simulink model "ActuatorModel"  (R2020a)
settings: Solver=VariableStepAuto  StartTime=0.0  StopTime=10.0  RelTol=1e-3
values from neighbouring files (symbols this model uses):
  SA_Gain = A_Max/X_Max    (= 16)    [ActuatorModelParams.m]
libraries: fl_lib x34, nesl_utility x4, sdl_lib x1, SignalEditorBlockLib x1
(part 2 of 2)

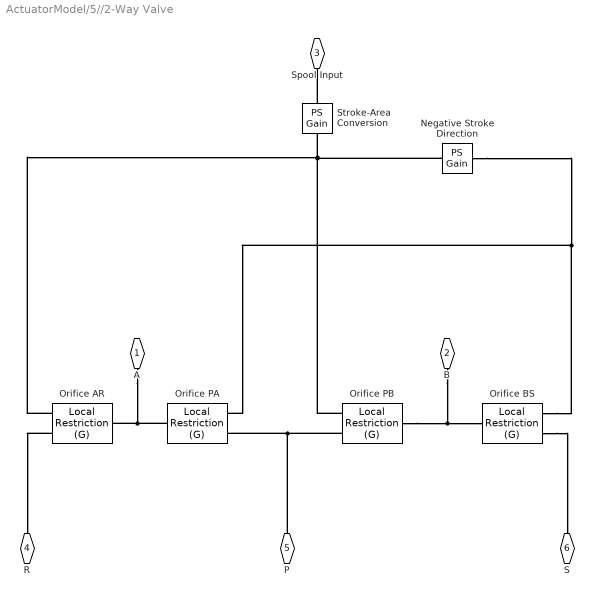
== system ActuatorModel/5//2-Way Valve ==
  Negative Stroke Direction : fl_lib/Physical Signals/Functions/PS Gain  gain=-1
  Orifice AR : fl_lib/Gas/Elements/Local Restriction (G)  restriction_type=foundation.enum.restriction_type.variable  restriction_area=1e-3 m^2  min_area=AR_MinArea in^2  max_area=AR_MaxArea mm^2  area=AR_OriArea in^2  Cd=AR_Cd  B_lam=0.999
      settings: SourceProductBaseCode=SS  InternalSimscapePortConfiguration="{\"Bottom\":[],\"Left\":[{\"id\":\"A\",\"label\":\"A\",\"type\":\"foundation.gas.gas\"},{\"id\":\"area_in\",\"label\":\"AR\",\"type\":\"input\"}],\"Right\":[{\"id\":\"B\",\"label\":\"B\",\"type\":\"foundation.gas.gas\"}],\"Top\":[]}"
  Orifice BS : fl_lib/Gas/Elements/Local Restriction (G)  restriction_type=foundation.enum.restriction_type.variable  restriction_area=1e-3 m^2  min_area=BS_MinArea in^2  max_area=BS_MaxArea mm^2  area=BS_OriArea in^2  Cd=BS_Cd  B_lam=0.999
      settings: SourceProductBaseCode=SS  InternalSimscapePortConfiguration="{\"Bottom\":[],\"Left\":[{\"id\":\"A\",\"label\":\"A\",\"type\":\"foundation.gas.gas\"},{\"id\":\"area_in\",\"label\":\"AR\",\"type\":\"input\"}],\"Right\":[{\"id\":\"B\",\"label\":\"B\",\"type\":\"foundation.gas.gas\"}],\"Top\":[]}"
  Orifice PA : fl_lib/Gas/Elements/Local Restriction (G)  restriction_type=foundation.enum.restriction_type.variable  restriction_area=1e-3 m^2  min_area=PA_MinArea in^2  max_area=PA_MaxArea mm^2  area=PA_OriArea in^2  Cd=PA_Cd  B_lam=0.999
      settings: SourceProductBaseCode=SS  InternalSimscapePortConfiguration="{\"Bottom\":[],\"Left\":[{\"id\":\"A\",\"label\":\"A\",\"type\":\"foundation.gas.gas\"},{\"id\":\"area_in\",\"label\":\"AR\",\"type\":\"input\"}],\"Right\":[{\"id\":\"B\",\"label\":\"B\",\"type\":\"foundation.gas.gas\"}],\"Top\":[]}"
  Orifice PB : fl_lib/Gas/Elements/Local Restriction (G)  restriction_type=foundation.enum.restriction_type.variable  restriction_area=1e-3 m^2  min_area=PB_MinArea in^2  max_area=PB_MaxArea mm^2  area=PB_OriArea in^2  Cd=PB_Cd  B_lam=0.999
      settings: SourceProductBaseCode=SS  InternalSimscapePortConfiguration="{\"Bottom\":[],\"Left\":[{\"id\":\"A\",\"label\":\"A\",\"type\":\"foundation.gas.gas\"},{\"id\":\"area_in\",\"label\":\"AR\",\"type\":\"input\"}],\"Right\":[{\"id\":\"B\",\"label\":\"B\",\"type\":\"foundation.gas.gas\"}],\"Top\":[]}"
  Stroke-Area Conversion : fl_lib/Physical Signals/Functions/PS Gain  gain=SA_Gain
  A : PMIOPort  Side=Left
  B : PMIOPort  Port=2  Side=Left
  Spool Input : PMIOPort  Port=3  Side=Left
  R : PMIOPort  Port=4  Side=Right
  P : PMIOPort  Port=5  Side=Right
  S : PMIOPort  Port=6  Side=Right
  connections:
  Orifice PA/RConn1 -- A/RConn1 -- Orifice AR/RConn1
  Negative Stroke Direction/RConn1 -- Orifice PA/LConn2 -- Orifice BS/LConn2
  Orifice BS/LConn1 -- S/RConn1
  Negative Stroke Direction/LConn1 -- Orifice PB/LConn2 -- Orifice AR/LConn2 -- Stroke-Area Conversion/RConn1
  Orifice PB/LConn1 -- Orifice PA/LConn1 -- P/RConn1
  Orifice PB/RConn1 -- B/RConn1 -- Orifice BS/RConn1
  Stroke-Area Conversion/LConn1 -- Spool Input/RConn1
  Orifice AR/LConn1 -- R/RConn1

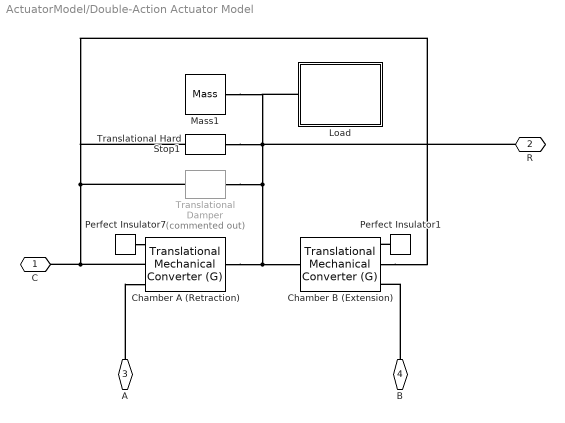
== system ActuatorModel/Double-Action Actuator Model ==
  Chamber A (Retraction) : fl_lib/Gas/Elements/Translational Mechanical Converter (G)  mech_orientation=simscape.enum.posneg.negative  interface_area=ChA_InterfaceArea in^2  length_init=ChA_InitialDisplacement in  dead_volume=ChA_DeadVol in^3  area_A=ChA_PortArea in^2  environment_spec=foundation.enum.pressure_spec.atmospheric  environment_pressure=0.101325 MPa  p_I_specify=off  p_I_priority=High  p_I=0.101325 MPa  p_I_nominal_specify=off  p_I_nominal_unit=MPa  p_I_nominal_value=1  T_I_specify=off  T_I_priority=High  T_I=293.15 K  T_I_nominal_specify=off  T_I_nominal_unit=K  T_I_nominal_value=1  rho_converter_specify=off  rho_converter_priority=None  rho_converter=1.2 kg/m^3  rho_converter_nominal_specify=off  rho_converter_nominal_unit=kg/m^3  rho_converter_nominal_value=1
      settings: SourceProductBaseCode=SS  InternalSimscapePortConfiguration="{\"Bottom\":[],\"Left\":[{\"id\":\"A\",\"label\":\"A\",\"type\":\"foundation.gas.gas\"},{\"id\":\"C\",\"label\":\"C\",\"type\":\"foundation.mechanical.translational.translational\"},{\"id\":\"H\",\"label\":\"H\",\"type\":\"foundation.thermal.thermal\"}],\"Right\":[{\"id\":\"R\",\"label\":\"R\",\"type\":\"foundation.mechanical.translational.translational\"}],\"Top\":[]}"
  Chamber B (Extension) : fl_lib/Gas/Elements/Translational Mechanical Converter (G)  mech_orientation=simscape.enum.posneg.positive  interface_area=ChB_InterfaceArea in^2  length_init=ChB_InitialDisplacement in  dead_volume=ChB_DeadVol in^3  area_A=ChB_PortArea m^2  environment_spec=foundation.enum.pressure_spec.atmospheric  environment_pressure=0.101325 MPa  p_I_specify=off  p_I_priority=High  p_I=0.101325 MPa  p_I_nominal_specify=off  p_I_nominal_unit=MPa  p_I_nominal_value=1  T_I_specify=off  T_I_priority=High  T_I=293.15 K  T_I_nominal_specify=off  T_I_nominal_unit=K  T_I_nominal_value=1  rho_converter_specify=off  rho_converter_priority=None  rho_converter=1.2 kg/m^3  rho_converter_nominal_specify=off  rho_converter_nominal_unit=kg/m^3  rho_converter_nominal_value=1
      settings: SourceProductBaseCode=SS  InternalSimscapePortConfiguration="{\"Bottom\":[],\"Left\":[{\"id\":\"A\",\"label\":\"A\",\"type\":\"foundation.gas.gas\"},{\"id\":\"C\",\"label\":\"C\",\"type\":\"foundation.mechanical.translational.translational\"},{\"id\":\"H\",\"label\":\"H\",\"type\":\"foundation.thermal.thermal\"}],\"Right\":[{\"id\":\"R\",\"label\":\"R\",\"type\":\"foundation.mechanical.translational.translational\"}],\"Top\":[]}"
  Load : Subsystem
  Mass1 : fl_lib/Mechanical/Translational Elements/Mass  mass=Actuator_RodMass kg  v_specify=off  v_priority=High  v=0 m/s  v_nominal_specify=off  v_nominal_unit=m/s  v_nominal_value=1  f_specify=off  f_priority=None  f=0 N  f_nominal_specify=off  f_nominal_unit=N  f_nominal_value=1
  Perfect Insulator1 : fl_lib/Thermal/Thermal Elements/Perfect Insulator  T_specify=off  T_priority=None  T=0 K  T_nominal_specify=off  T_nominal_unit=K  T_nominal_value=1
  Perfect Insulator7 : fl_lib/Thermal/Thermal Elements/Perfect Insulator  T_specify=off  T_priority=None  T=0 K  T_nominal_specify=off  T_nominal_unit=K  T_nominal_value=1
  Translational Damper : sdl_lib/Couplings & Drives/Springs & Dampers/Translational Damper  Commented=on  D=100 lbf/(in/s)  enable_faults=0  b_fault=1e6 N/(m/s)  temporal_fault=0  fault_time=5 s  shock_fault=0  acceleration_limit=100 m/s^2  shock_limit=1  report_fault=1
      settings: SourceProductBaseCode=LD
  Translational Hard Stop1 : fl_lib/Mechanical/Translational Elements/Translational Hard Stop  upper_bnd=Actuator_StopU in  lower_bnd=Actuator_StopL in  stiff_up=1e7 N/m  stiff_low=1e7 N/m  D_up=150000 N/(m/s)  D_low=150000 N/(m/s)  model=simscape.enum.hardstop.fulldamped  transition=0.1 mm  v_specify=off  v_priority=None  v=0 m/s  v_nominal_specify=off  v_nominal_unit=m/s  v_nominal_value=1  f_specify=off  f_priority=None  f=0 N  f_nominal_specify=off  f_nominal_unit=N  f_nominal_value=1  x_specify=off  x_priority=High  x=0 m  x_nominal_specify=off  x_nominal_unit=m  x_nominal_value=1
  C : PMIOPort  Side=Left
  R : PMIOPort  Port=2  Side=Right
  A : PMIOPort  Port=3  Side=Right
  B : PMIOPort  Port=4  Side=Right
  connections:
  Chamber A (Retraction)/RConn1 -- Translational Damper/LConn1 -- R/RConn1 -- Load/LConn1 -- Mass1/LConn1 -- Translational Hard Stop1/LConn1 -- Chamber B (Extension)/RConn1
  A/RConn1 -- Chamber A (Retraction)/LConn1
  Perfect Insulator7/LConn1 -- Chamber A (Retraction)/LConn3
  Chamber A (Retraction)/LConn2 -- C/RConn1 -- Translational Damper/RConn1 -- Translational Hard Stop1/RConn1 -- Chamber B (Extension)/LConn2
  Perfect Insulator1/LConn1 -- Chamber B (Extension)/LConn3
  B/RConn1 -- Chamber B (Extension)/LConn1

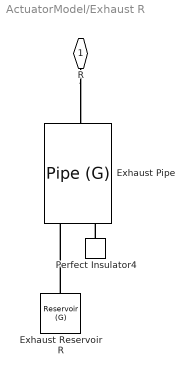
== system ActuatorModel/Exhaust R ==
  Exhaust Pipe : fl_lib/Gas/Elements/Pipe (G)  length=ExhPR_Length in  area=ExhPR_Area in^2  Dh=ExhPR_HDiam in  length_add=0.1 m  roughness=15e-6 m  Re_lam=2000  Re_tur=4000  shape_factor=64  Nu_lam=3.66  p_I_specify=off  p_I_priority=High  p_I=0.101325 MPa  p_I_nominal_specify=off  p_I_nominal_unit=MPa  p_I_nominal_value=1  T_I_specify=off  T_I_priority=High  T_I=293.15 K  T_I_nominal_specify=off  T_I_nominal_unit=K  T_I_nominal_value=1  rho_pipe_specify=off  rho_pipe_priority=None  rho_pipe=1.2 kg/m^3  rho_pipe_nominal_specify=off  rho_pipe_nominal_unit=kg/m^3  rho_pipe_nominal_value=1
      settings: SourceProductBaseCode=SS
  Exhaust Reservoir R : fl_lib/Gas/Elements/Reservoir (G)  pressure_spec=foundation.enum.pressure_spec.specified  reservoir_pressure=ExhRR_Pres atm  reservoir_temperature=ExhRR_Temp K  area_A=ExhRR_Area in^2
      settings: SourceProductBaseCode=SS
  Perfect Insulator4 : fl_lib/Thermal/Thermal Elements/Perfect Insulator  T_specify=off  T_priority=None  T=0 K  T_nominal_specify=off  T_nominal_unit=K  T_nominal_value=1
  R : PMIOPort  Side=Right
  connections:
  Perfect Insulator4/LConn1 -- Exhaust Pipe/LConn2
  R/RConn1 -- Exhaust Pipe/RConn1
  Exhaust Reservoir R/LConn1 -- Exhaust Pipe/LConn1

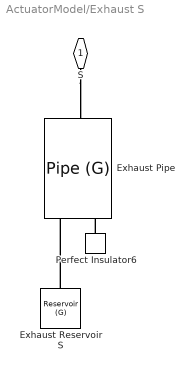
== system ActuatorModel/Exhaust S ==
  Exhaust Pipe : fl_lib/Gas/Elements/Pipe (G)  length=ExhPS_Length in  area=ExhPS_Area in^2  Dh=ExhPS_HDiam in  length_add=0.1 m  roughness=15e-6 m  Re_lam=2000  Re_tur=4000  shape_factor=64  Nu_lam=3.66  p_I_specify=off  p_I_priority=High  p_I=0.101325 MPa  p_I_nominal_specify=off  p_I_nominal_unit=MPa  p_I_nominal_value=1  T_I_specify=off  T_I_priority=High  T_I=293.15 K  T_I_nominal_specify=off  T_I_nominal_unit=K  T_I_nominal_value=1  rho_pipe_specify=off  rho_pipe_priority=None  rho_pipe=1.2 kg/m^3  rho_pipe_nominal_specify=off  rho_pipe_nominal_unit=kg/m^3  rho_pipe_nominal_value=1
      settings: SourceProductBaseCode=SS
  Exhaust Reservoir S : fl_lib/Gas/Elements/Reservoir (G)  pressure_spec=foundation.enum.pressure_spec.specified  reservoir_pressure=ExhRS_Pres atm  reservoir_temperature=ExhRS_Temp K  area_A=ExhRS_Area in^2
      settings: SourceProductBaseCode=SS
  Perfect Insulator6 : fl_lib/Thermal/Thermal Elements/Perfect Insulator  T_specify=off  T_priority=None  T=0 K  T_nominal_specify=off  T_nominal_unit=K  T_nominal_value=1
  S : PMIOPort  Side=Right
  connections:
  Perfect Insulator6/LConn1 -- Exhaust Pipe/LConn2
  S/RConn1 -- Exhaust Pipe/RConn1
  Exhaust Reservoir S/LConn1 -- Exhaust Pipe/LConn1

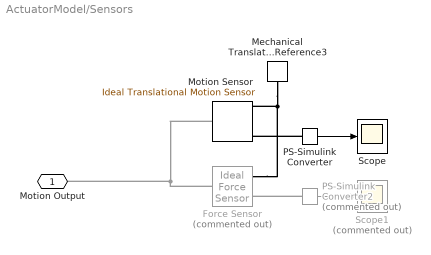
== system ActuatorModel/Sensors ==
  Force Sensor : fl_lib/Mechanical/Mechanical Sensors/Ideal Force Sensor  Commented=on
  Mechanical Translational Reference3 : fl_lib/Mechanical/Translational Elements/Mechanical Translational Reference
  Motion Sensor : fl_lib/Mechanical/Mechanical Sensors/Ideal Translational Motion Sensor  offset=0 in
  PS-Simulink Converter : nesl_utility/PS-Simulink Converter  PhysicalDomain=network_engine_domain  SubClassName=ps_output  LeftPortType=input  RightPortType=output  PseudoPeriodic=off  Frequencies=[]  Unit=in  AffineConversion=off
  PS-Simulink Converter2 : nesl_utility/PS-Simulink Converter  Commented=on  PhysicalDomain=network_engine_domain  SubClassName=ps_output  LeftPortType=input  RightPortType=output  PseudoPeriodic=off  Frequencies=[]  Unit=inherit  AffineConversion=off
  Scope : Scope
  Scope1 : Scope  Commented=on
  Motion Output : PMIOPort  Side=Left
  wires:
  PS-Simulink Converter2/1 -> Scope1/1
  PS-Simulink Converter/1 -> Scope/1
  connections:
  Force Sensor/LConn1 -- Motion Sensor/LConn1 -- Motion Output/RConn1
  PS-Simulink Converter/LConn1 -- Motion Sensor/RConn3
  Mechanical Translational Reference3/LConn1 -- Force Sensor/RConn1 -- Motion Sensor/RConn1
  PS-Simulink Converter2/LConn1 -- Force Sensor/RConn2

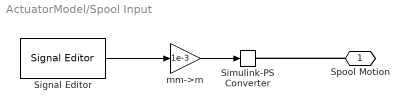
== system ActuatorModel/Spool Input ==
  Signal Editor : SignalEditorBlockLib/Signal Editor  FileName=2PulseScenario.mat  ActiveScenario=Scenario  ActiveSignal=Signal 1  IsBus=off  OutputBusObjectStr=Bus: BusObject  SampleTime=0  Interpolate=off  ZeroCross=off  OutputAfterFinalValue=Setting to zero  Unit=inherit  PreserveSignalName=on
  Simulink-PS Converter : nesl_utility/Simulink-PS Converter  PhysicalDomain=network_engine_domain  SubClassName=ps_input  LeftPortType=input  RightPortType=output  PseudoPeriodic=off  Frequencies=[]  NoiseDistribution=none  NoiseParameters=[]  Unit=1  AffineConversion=off  FilteringAndDerivatives=provide  SimscapeFilterOrder=1  InputFilterTimeConstant=0.001  UdotUserProvided=0
  mm->m : Gain  Gain=1e-3
  Spool Motion : PMIOPort  Side=Right
  wires:
  mm->m/1 -> Simulink-PS Converter/1
  Signal Editor/1 -> mm->m/1
  connections:
  Spool Motion/RConn1 -- Simulink-PS Converter/RConn1

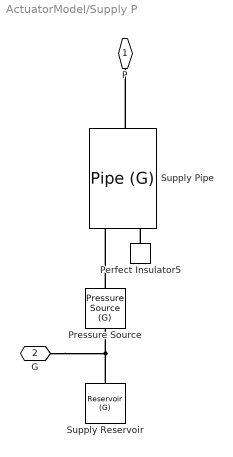
== system ActuatorModel/Supply P ==
  Perfect Insulator5 : fl_lib/Thermal/Thermal Elements/Perfect Insulator  T_specify=off  T_priority=None  T=0 K  T_nominal_specify=off  T_nominal_unit=K  T_nominal_value=1
  Pressure Source : fl_lib/Gas/Sources/Pressure Source (G)  power_spec=foundation.enum.power_spec.isentropic  pressure_differential=SupPS_Diff psi  area_A=SupPS_AreaA in^2  area_B=SupPS_AreaB in^2
      settings: SourceProductBaseCode=SS  InternalSimscapePortConfiguration="{\"Bottom\":[],\"Left\":[{\"id\":\"A\",\"label\":\"A\",\"type\":\"foundation.gas.gas\"}],\"Right\":[{\"id\":\"B\",\"label\":\"B\",\"type\":\"foundation.gas.gas\"}],\"Top\":[]}"
  Supply Pipe : fl_lib/Gas/Elements/Pipe (G)  length=SupPP_Length in  area=SupPP_Area in^2  Dh=SupPP_HDiam in  length_add=0.1 m  roughness=15e-6 m  Re_lam=2000  Re_tur=4000  shape_factor=64  Nu_lam=3.66  p_I_specify=off  p_I_priority=High  p_I=0.101325 MPa  p_I_nominal_specify=off  p_I_nominal_unit=MPa  p_I_nominal_value=1  T_I_specify=off  T_I_priority=High  T_I=293.15 K  T_I_nominal_specify=off  T_I_nominal_unit=K  T_I_nominal_value=1  rho_pipe_specify=off  rho_pipe_priority=None  rho_pipe=1.2 kg/m^3  rho_pipe_nominal_specify=off  rho_pipe_nominal_unit=kg/m^3  rho_pipe_nominal_value=1
      settings: SourceProductBaseCode=SS
  Supply Reservoir : fl_lib/Gas/Elements/Reservoir (G)  pressure_spec=foundation.enum.pressure_spec.specified  reservoir_pressure=SupRP_Pres atm  reservoir_temperature=SupRP_Temp K  area_A=SupRP_Area in^2
      settings: SourceProductBaseCode=SS
  P : PMIOPort  Side=Right
  G : PMIOPort  Port=2  Side=Left
  connections:
  Pressure Source/RConn1 -- Supply Pipe/LConn1
  Supply Reservoir/LConn1 -- G/RConn1 -- Pressure Source/LConn1
  Perfect Insulator5/LConn1 -- Supply Pipe/LConn2
  Supply Pipe/RConn1 -- P/RConn1

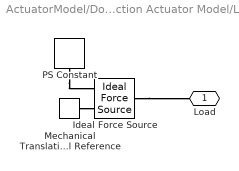
== system ActuatorModel/Double-Action Actuator Model/Load ==
  Ideal Force Source : fl_lib/Mechanical/Mechanical Sources/Ideal Force Source
  Mechanical Translational Reference : fl_lib/Mechanical/Translational Elements/Mechanical Translational Reference
  PS Constant : fl_lib/Physical Signals/Sources/PS Constant  constant=Const_Load lbf
  Load : PMIOPort  Side=Left
  connections:
  PS Constant/RConn1 -- Ideal Force Source/RConn1
  Mechanical Translational Reference/LConn1 -- Ideal Force Source/RConn2
  Ideal Force Source/LConn1 -- Load/RConn1
